simulink model "ROBOTIC_ARM_sim"  (R2024b)
settings: Solver=VariableStepAuto  StartTime=0.0  StopTime=5  RelTol=1e-3
model workspace: external: MATLAB File D:\Vaults\Mechatronic Systems Design Project\Arm\Control\robotic_arm_4dof_matlab\scripts\initalize_model.m (data not in the file)
undefined symbols (not defined in the file): cubes, sim_relative, smiData, v_b, X, Y, Z
libraries: sm_lib x75, nesl_utility x10, BUMBLEBEE x8
(part 1 of 2)
settings Model: Creator=Mohammed Hany  LastModifiedBy=Mohammed Hany

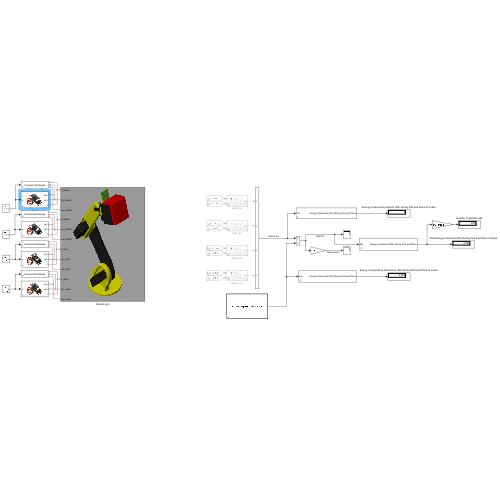
[thumbnail: Simulink's stored preview of the top-level diagram]
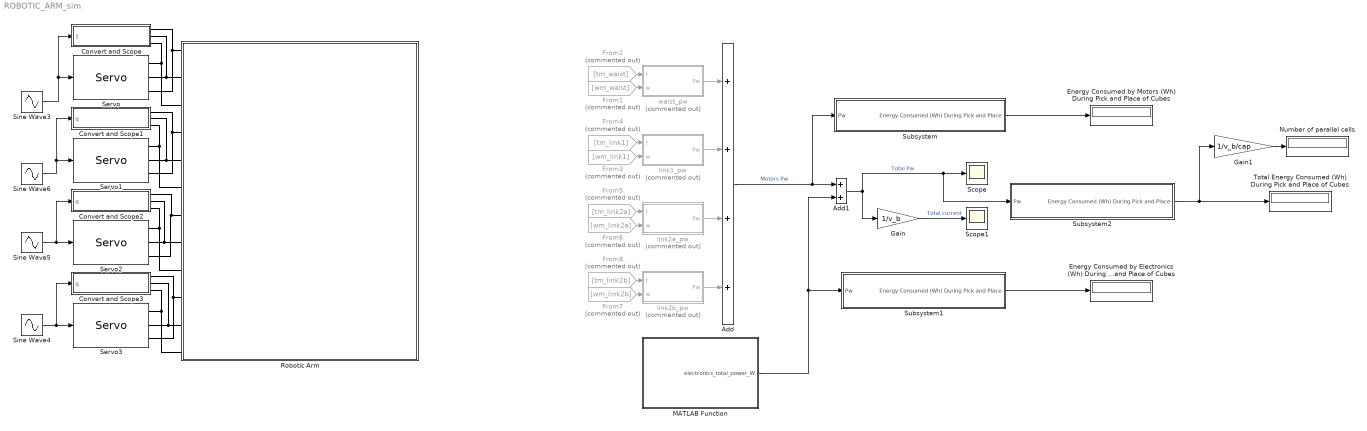
== system ROBOTIC_ARM_sim ==
  Add : Sum  Inputs=++++
  Add1 : Sum
  Convert and Scope : Subsystem  ReferencedSubsystem=convert_and_scope
      settings: PortSchema="{\"entries\":[{\"content\":{\"sides\":[{\"content\":{\"connectorIds\":[\"LConn1\",\"LConn2\"]},\"type\":\"ConnectorPlacement.EquallySpacedRectSide\",\"uuid\":\"e9d3fa8a-a658-421c-a715-dee0f5d0277a\"},{\"content\":{\"side\":\"RIGHT\"},\"type\":\"ConnectorPlacement.EquallySpacedRectSide\",\"uuid\":\"8f4733ec-a2c9-48cc-bea1-8566252d8d79\"},{\"content\":{\"connectorIds\":[\"In1\"],\"side\":\"TOP\"},\"type\":\"ConnectorPlacement.EquallySpacedRectSide\",\"uuid\":\"ce7ba2ac-a2b1-42d2-bf3f-12c1e6573af0\"},{\"content\":{\"connectorIds\":[\"RConn1\",\"RConn2\",\"RConn3\"],\"side\":\"BOTTOM\"},\"type\":\"ConnectorPlacement.EquallySpacedRectSide\",\"uuid\":\"8390652c-32f7-42bc-a6e4-5fbde262c394\"}]},\"type\":\"ConnectorPlacement.EquallySpacedConnector\",\"uuid\":\"90170afb-acac-48c1-856c-2f07de9489fa\"}],\"packageUris\":[\"http://schema.mathworks.com/mf0/Connector/R2020b\"],\"version\":\"1.0\"}"
  Convert and Scope1 : Subsystem  mask(Tool){}
      mask help: Takes the input angular position, measured angular position, measured angular velocity, torque, current, and voltage. It converts them to simulink signals and displays them on a scope. It uses a GOTO tag to cleanly expose torque, angular velocity, current, and voltage for furter computations in this model
      settings: PortSchema="{\"entries\":[{\"content\":{\"sides\":[{\"content\":{},\"type\":\"ConnectorPlacement.EquallySpacedRectSide\",\"uuid\":\"e9d3fa8a-a658-421c-a715-dee0f5d0277a\"},{\"content\":{\"side\":\"RIGHT\"},\"type\":\"ConnectorPlacement.EquallySpacedRectSide\",\"uuid\":\"8f4733ec-a2c9-48cc-bea1-8566252d8d79\"},{\"content\":{\"connectorIds\":[\"In1\"],\"side\":\"TOP\"},\"type\":\"ConnectorPlacement.EquallySpacedRectSide\",\"uuid\":\"ce7ba2ac-a2b1-42d2-bf3f-12c1e6573af0\"},{\"content\":{\"connectorIds\":[\"RConn1\",\"RConn2\",\"RConn3\"],\"side\":\"BOTTOM\"},\"type\":\"ConnectorPlacement.EquallySpacedRectSide\",\"uuid\":\"8390652c-32f7-42bc-a6e4-5fbde262c394\"}]},\"type\":\"ConnectorPlacement.EquallySpacedConnector\",\"uuid\":\"90170afb-acac-48c1-856c-2f07de9489fa\"}],\"packageUris\":[\"http://schema.mathworks.com/mf0/Connector/R2020b\"],\"version\":\"1.0\"}"
      mask Display: disp('Convert and Scope');
  Convert and Scope2 : Subsystem  mask(Tool){}
      mask help: Takes the input angular position, measured angular position, measured angular velocity, torque, current, and voltage. It converts them to simulink signals and displays them on a scope. It uses a GOTO tag to cleanly expose torque, angular velocity, current, and voltage for furter computations in this model
      settings: PortSchema="{\"entries\":[{\"content\":{\"sides\":[{\"content\":{},\"type\":\"ConnectorPlacement.EquallySpacedRectSide\",\"uuid\":\"e9d3fa8a-a658-421c-a715-dee0f5d0277a\"},{\"content\":{\"side\":\"RIGHT\"},\"type\":\"ConnectorPlacement.EquallySpacedRectSide\",\"uuid\":\"8f4733ec-a2c9-48cc-bea1-8566252d8d79\"},{\"content\":{\"connectorIds\":[\"In1\"],\"side\":\"TOP\"},\"type\":\"ConnectorPlacement.EquallySpacedRectSide\",\"uuid\":\"ce7ba2ac-a2b1-42d2-bf3f-12c1e6573af0\"},{\"content\":{\"connectorIds\":[\"RConn1\",\"RConn2\",\"RConn3\"],\"side\":\"BOTTOM\"},\"type\":\"ConnectorPlacement.EquallySpacedRectSide\",\"uuid\":\"8390652c-32f7-42bc-a6e4-5fbde262c394\"}]},\"type\":\"ConnectorPlacement.EquallySpacedConnector\",\"uuid\":\"90170afb-acac-48c1-856c-2f07de9489fa\"}],\"packageUris\":[\"http://schema.mathworks.com/mf0/Connector/R2020b\"],\"version\":\"1.0\"}"
      mask Display: disp('Convert and Scope');
  Convert and Scope3 : Subsystem  mask(Tool){}
      mask help: Takes the input angular position, measured angular position, measured angular velocity, torque, current, and voltage. It converts them to simulink signals and displays them on a scope. It uses a GOTO tag to cleanly expose torque, angular velocity, current, and voltage for furter computations in this model
      settings: PortSchema="{\"entries\":[{\"content\":{\"sides\":[{\"content\":{},\"type\":\"ConnectorPlacement.EquallySpacedRectSide\",\"uuid\":\"e9d3fa8a-a658-421c-a715-dee0f5d0277a\"},{\"content\":{\"side\":\"RIGHT\"},\"type\":\"ConnectorPlacement.EquallySpacedRectSide\",\"uuid\":\"8f4733ec-a2c9-48cc-bea1-8566252d8d79\"},{\"content\":{\"connectorIds\":[\"In1\"],\"side\":\"TOP\"},\"type\":\"ConnectorPlacement.EquallySpacedRectSide\",\"uuid\":\"ce7ba2ac-a2b1-42d2-bf3f-12c1e6573af0\"},{\"content\":{\"connectorIds\":[\"RConn1\",\"RConn2\",\"RConn3\"],\"side\":\"BOTTOM\"},\"type\":\"ConnectorPlacement.EquallySpacedRectSide\",\"uuid\":\"8390652c-32f7-42bc-a6e4-5fbde262c394\"}]},\"type\":\"ConnectorPlacement.EquallySpacedConnector\",\"uuid\":\"90170afb-acac-48c1-856c-2f07de9489fa\"}],\"packageUris\":[\"http://schema.mathworks.com/mf0/Connector/R2020b\"],\"version\":\"1.0\"}"
      mask Display: disp('Convert and Scope');
  Energy Consumed by Electronics (Wh) During Pick and Place of Cubes : Display
  Energy Consumed by Motors (Wh) During Pick and Place of Cubes : Display
  From1 : From  Commented=on  GotoTag=wm_waist
  From2 : From  Commented=on  GotoTag=tm_waist
  From3 : From  Commented=on  GotoTag=wm_link1
  From4 : From  Commented=on  GotoTag=tm_link1
  From5 : From  Commented=on  GotoTag=tm_link2a
  From6 : From  Commented=on  GotoTag=wm_link2a
  From7 : From  Commented=on  GotoTag=wm_link2b
  From8 : From  Commented=on  GotoTag=tm_link2b
  Gain : Gain  Gain=1/v_b
  Gain1 : Gain  Gain=1/v_b/cap
  MATLAB Function : MATLAB Function  TreatAsAtomicUnit=on
  Number of parallel cells : Display
  Robotic Arm : Subsystem
      mask Display: image('isometric.png');
  Scope : Scope
  Scope1 : Scope
  Servo{,1..3} (4 alike) : BUMBLEBEE/Servo  J=0 cm^2*g  La=12e-6 H  P_rated=4.2 W  V_i_noload=6 V  V_rated=6 V  i_noload=0.05 A  w_max=99 rpm  w_rated=71.43 rpm  ratio=1
  Sine Wave3 : Sin  Amplitude=55  Bias=30  SampleTime=0
  Sine Wave4 : Sin  Amplitude=180  SampleTime=0
  Sine Wave5 : Sin  Amplitude=100  Bias=-50  SampleTime=0
  Sine Wave6 : Sin  Amplitude=100  Bias=50  SampleTime=0
  Subsystem : Subsystem  mask{cubes=cubes}
      mask prompts: cubes "Number of cubes for pick and place"
  Subsystem1 : Subsystem  mask{cubes=cubes}
      mask prompts: cubes "Number of cubes for pick and place"
  Subsystem2 : Subsystem  mask{cubes=cubes}
      mask prompts: cubes "Number of cubes for pick and place"
  Total Energy Consumed (Wh) During Pick and Place of Cubes : Display
  link1_pw : Subsystem  Commented=on
  link2a_pw : Subsystem  Commented=on
  link2b_pw : Subsystem  Commented=on
  waist_pw : Subsystem  Commented=on
  wires:
  link2b_pw/1(Pw) -> Add/4
  link1_pw/1(Pw) -> Add/2
  waist_pw/1(Pw) -> Add/1
  Add/1 -> Subsystem/1(Pw), Add1/1  "Motors Pw"
  Subsystem1/1(Energy Consumed (Wh) During Pick and Place) -> Energy Consumed by Electronics (Wh) During Pick and Place of Cubes/1
  MATLAB Function/1(electronics_total_power_W) -> Add1/2, Subsystem1/1(Pw)
  Subsystem/1(Energy Consumed (Wh) During Pick and Place) -> Energy Consumed by Motors (Wh) During Pick and Place of Cubes/1
  Gain/1 -> Scope1/1  "Total current"
  Add1/1 -> Gain/1, Subsystem2/1(Pw), Scope/1  "Total Pw"
  Subsystem2/1(Energy Consumed (Wh) During Pick and Place) -> Gain1/1, Total Energy Consumed (Wh) During Pick and Place of Cubes/1
  Gain1/1 -> Number of parallel cells/1
  link2a_pw/1(Pw) -> Add/3
  Sine Wave3/1 -> Convert and Scope/1, Servo/1
  From1/1 -> waist_pw/2(w)
  From2/1 -> waist_pw/1(t)
  From4/1 -> link1_pw/1(t)
  From3/1 -> link1_pw/2(w)
  From5/1 -> link2a_pw/1(t)
  From6/1 -> link2a_pw/2(w)
  From7/1 -> link2b_pw/2(w)
  From8/1 -> link2b_pw/1(t)
  Sine Wave6/1 -> Convert and Scope1/1(q), Servo1/1
  Sine Wave5/1 -> Convert and Scope2/1(q), Servo2/1
  Sine Wave4/1 -> Convert and Scope3/1(q), Servo3/1
  connections:
  Servo/RConn2 -- Convert and Scope/RConn2 -- Robotic Arm/LConn2
  Servo/RConn1 -- Convert and Scope/RConn1 -- Robotic Arm/LConn3
  Servo1/RConn2 -- Convert and Scope1/RConn2 -- Robotic Arm/LConn5
  Servo1/RConn1 -- Convert and Scope1/RConn1 -- Robotic Arm/LConn6
  Servo1/RConn3 -- Convert and Scope1/RConn3 -- Robotic Arm/LConn4
  Servo2/RConn2 -- Convert and Scope2/RConn2 -- Robotic Arm/LConn8
  Servo2/RConn1 -- Robotic Arm/LConn9 -- Convert and Scope2/RConn1
  Servo2/RConn3 -- Convert and Scope2/RConn3 -- Robotic Arm/LConn7
  Servo3/RConn2 -- Convert and Scope3/RConn2 -- Robotic Arm/LConn11
  Servo3/RConn1 -- Convert and Scope3/RConn1 -- Robotic Arm/LConn12
  Servo3/RConn3 -- Convert and Scope3/RConn3 -- Robotic Arm/LConn10
  Servo/RConn3 -- Convert and Scope/RConn3 -- Robotic Arm/LConn1

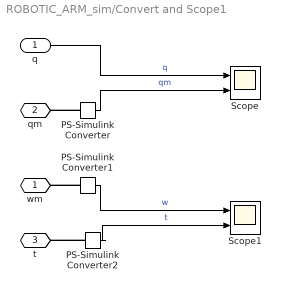
== system ROBOTIC_ARM_sim/Convert and Scope1 ==
  q : Inport
  PS-Simulink Converter : nesl_utility/PS-Simulink Converter  PhysicalDomain=network_engine_domain  SubClassName=ps_output  LeftPortType=input  RightPortType=output  PseudoPeriodic=off  Frequencies=[]  VectorFormat=inherit  Unit=deg  AffineConversion=off
  PS-Simulink Converter1 : nesl_utility/PS-Simulink Converter  PhysicalDomain=network_engine_domain  SubClassName=ps_output  LeftPortType=input  RightPortType=output  PseudoPeriodic=off  Frequencies=[]  VectorFormat=inherit  Unit=rpm  AffineConversion=off
  PS-Simulink Converter2 : nesl_utility/PS-Simulink Converter  PhysicalDomain=network_engine_domain  SubClassName=ps_output  LeftPortType=input  RightPortType=output  PseudoPeriodic=off  Frequencies=[]  VectorFormat=inherit  Unit=N*m  AffineConversion=off
  Scope : Scope  NumInputPorts=2
  Scope1 : Scope  NumInputPorts=2
  wm : PMIOPort  Side=Right
  qm : PMIOPort  Port=2  Side=Right
  t : PMIOPort  Port=3  Side=Right
  wires:
  q/1 -> Scope/1  "q"
  PS-Simulink Converter/1 -> Scope/2  "qm"
  PS-Simulink Converter2/1 -> Scope1/2  "t"
  PS-Simulink Converter1/1 -> Scope1/1  "w"
  connections:
  PS-Simulink Converter1/LConn1 -- wm/RConn1
  PS-Simulink Converter/LConn1 -- qm/RConn1
  PS-Simulink Converter2/LConn1 -- t/RConn1

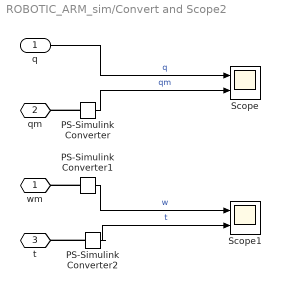
== system ROBOTIC_ARM_sim/Convert and Scope2 ==
  q : Inport
  PS-Simulink Converter : nesl_utility/PS-Simulink Converter  PhysicalDomain=network_engine_domain  SubClassName=ps_output  LeftPortType=input  RightPortType=output  PseudoPeriodic=off  Frequencies=[]  VectorFormat=inherit  Unit=deg  AffineConversion=off
  PS-Simulink Converter1 : nesl_utility/PS-Simulink Converter  PhysicalDomain=network_engine_domain  SubClassName=ps_output  LeftPortType=input  RightPortType=output  PseudoPeriodic=off  Frequencies=[]  VectorFormat=inherit  Unit=rpm  AffineConversion=off
  PS-Simulink Converter2 : nesl_utility/PS-Simulink Converter  PhysicalDomain=network_engine_domain  SubClassName=ps_output  LeftPortType=input  RightPortType=output  PseudoPeriodic=off  Frequencies=[]  VectorFormat=inherit  Unit=N*m  AffineConversion=off
  Scope : Scope  NumInputPorts=2
  Scope1 : Scope  NumInputPorts=2
  wm : PMIOPort  Side=Right
  qm : PMIOPort  Port=2  Side=Right
  t : PMIOPort  Port=3  Side=Right
  wires:
  q/1 -> Scope/1  "q"
  PS-Simulink Converter/1 -> Scope/2  "qm"
  PS-Simulink Converter2/1 -> Scope1/2  "t"
  PS-Simulink Converter1/1 -> Scope1/1  "w"
  connections:
  PS-Simulink Converter1/LConn1 -- wm/RConn1
  PS-Simulink Converter/LConn1 -- qm/RConn1
  PS-Simulink Converter2/LConn1 -- t/RConn1

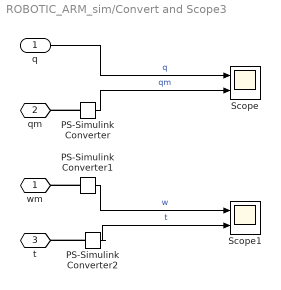
== system ROBOTIC_ARM_sim/Convert and Scope3 ==
  q : Inport
  PS-Simulink Converter : nesl_utility/PS-Simulink Converter  PhysicalDomain=network_engine_domain  SubClassName=ps_output  LeftPortType=input  RightPortType=output  PseudoPeriodic=off  Frequencies=[]  VectorFormat=inherit  Unit=deg  AffineConversion=off
  PS-Simulink Converter1 : nesl_utility/PS-Simulink Converter  PhysicalDomain=network_engine_domain  SubClassName=ps_output  LeftPortType=input  RightPortType=output  PseudoPeriodic=off  Frequencies=[]  VectorFormat=inherit  Unit=rpm  AffineConversion=off
  PS-Simulink Converter2 : nesl_utility/PS-Simulink Converter  PhysicalDomain=network_engine_domain  SubClassName=ps_output  LeftPortType=input  RightPortType=output  PseudoPeriodic=off  Frequencies=[]  VectorFormat=inherit  Unit=N*m  AffineConversion=off
  Scope : Scope  NumInputPorts=2
  Scope1 : Scope  NumInputPorts=2
  wm : PMIOPort  Side=Right
  qm : PMIOPort  Port=2  Side=Right
  t : PMIOPort  Port=3  Side=Right
  wires:
  q/1 -> Scope/1  "q"
  PS-Simulink Converter/1 -> Scope/2  "qm"
  PS-Simulink Converter2/1 -> Scope1/2  "t"
  PS-Simulink Converter1/1 -> Scope1/1  "w"
  connections:
  PS-Simulink Converter1/LConn1 -- wm/RConn1
  PS-Simulink Converter/LConn1 -- qm/RConn1
  PS-Simulink Converter2/LConn1 -- t/RConn1

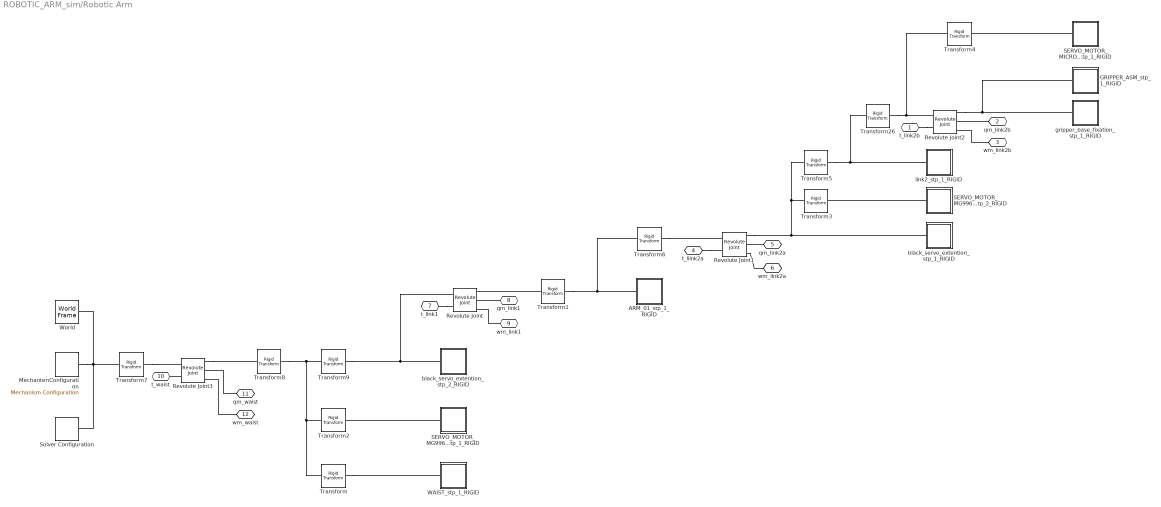
== system ROBOTIC_ARM_sim/Robotic Arm ==
  ARM_01_stp_1_RIGID : Subsystem
  GRIPPER_ASM_stp_1_RIGID : Subsystem
  MechanismConfiguration : sm_lib/Utilities/Mechanism Configuration  UniformGravity=Constant  GravityVector=[0 0 0]  GravityVectorUnits=m/s^2  LinearizationDelta=0.001  JointModeTransitionNonlinearIterations=2
  Revolute Joint{,1..3} (4 alike) : sm_lib/Joints/Revolute Joint  JointMode=Normal  CompositeWrenchDir=FollowerOnBase  CompositeWrenchFrame=BaseFrame  SenseConstraintForce=off  SenseConstraintTorque=off  SenseTotalForce=off  SenseTotalTorque=off  PositionTargetSpecify=off  PositionTargetPriority=High  PositionTargetValue=0  PositionTargetValueUnits=deg  VelocityTargetSpecify=off  VelocityTargetPriority=High  VelocityTargetValue=0  VelocityTargetValueUnits=deg/s  EquilibriumPosition=0  EquilibriumPositionUnits=deg  SpringStiffness=0  SpringStiffnessUnits=N*m/deg  DampingCoefficient=0  DampingCoefficientUnits=N*m/(deg/s)  LowerLimitSpecify=off  LowerLimitBound=-90  LowerLimitBoundUnits=deg  LowerLimitStiffness=1e4  LowerLimitStiffnessUnits=N*m/deg  LowerLimitDamping=10  LowerLimitDampingUnits=N*m/(deg/s)  LowerLimitTransitionRegionWidth=0.1  LowerLimitTransitionRegionWidthUnits=deg  UpperLimitSpecify=off  UpperLimitBound=90  UpperLimitBoundUnits=deg  UpperLimitStiffness=1e4  UpperLimitStiffnessUnits=N*m/deg  UpperLimitDamping=10  UpperLimitDampingUnits=N*m/(deg/s)  UpperLimitTransitionRegionWidth=0.1  UpperLimitTransitionRegionWidthUnits=deg  TorqueActuationMode=InputTorque  MotionActuationMode=ComputedMotion  SensePosition=on  SenseVelocity=on  SenseAcceleration=off  SenseTorqueForce=off  SenseLowerLimitTorqueForce=off  SenseUpperLimitTorqueForce=off
  SERVO_MOTOR_MG996R_stp_1_RIGID : Subsystem
  SERVO_MOTOR_MG996R_stp_2_RIGID : Subsystem
  SERVO_MOTOR_MICRO_9G_stp_1_RIGID : Subsystem
  Solver Configuration : nesl_utility/Solver Configuration  PhysicalDomain=network_engine_domain  SubClassName=solver  LeftPortType=input  RightPortType=generic  Tones=[]  Harmonics=[]  SimulateNoise=off  Profile=off  UseLocalSampling=off  EnableSwitchedLinearOptims=on  FrequencyDomain=off  UseCCode=off  RelTol=0.001  AbsTol=0.001  MinStep=1e-09  ToWorkspace=off  RevertToSquareIcSolve=off  NumHomotopyIterations=100  PhasorMode=off  PhasorModeNumHarmonics=1  ConsistencySolver=NEWTON_XTOL_AFTER_FTOL  IndexReductionMethod=DerivativeReplacement  DoDC=off  ResidualTolerance=1e-09  ConsistencyTolSource=GLOBAL  ConsistencyAbsTol=0.001  ConsistencyRelTol=0.001  ConsistencyTolFactor=0.001  UseLocalSolver=off  LocalSolverChoice=NE_BACKWARD_EULER_ADVANCER  ResolveIndetEquations=on  FunctionEvalNumThread=1  LocalSolverSampleTime=0.001  DoFixedCost=off  MaxNonlinIter=3  MaxModeIter=2  ComputeImpulses=off  ImpulseIterations=2  LinearAlgebra=auto  LinearAlgebraNumThread=0  EquationFormulation=NE_TIME_EF  DelaysMemoryBudget=1024  AutomaticFiltering=on  FilteringTimeConstant=0.001  PartitionStorageMethod=AS_NEEDED  PartitionMemoryBudget=1024  PartitionMethod=ROBUST  MultibodyUseLocalSolver=off  MultibodyLocalSolverChoice=ODE1  MultibodyLocalSolverSampleTime=0.001
  Transform : sm_lib/Frames and Transforms/Rigid Transform  RotationMethod=ArbitraryAxis  FollAlignAxisA=+X  BaseAlignAxisA=+Y  FollAlignAxisB=+Y  BaseAlignAxisB=+Z  RotationStandardAxis=+Z  RotationAngle=smiData.RigidTransform(25).angle  RotationAngleUnits=rad  RotationArbitraryAxis=smiData.RigidTransform(25).axis  RotationSequenceAxes=FollowerAxes  RotationSequence=XYX  RotationSequenceAngles=[0 0 0]  RotationSequenceAnglesUnits=deg  RotationMatrix=[1 0 0;0 1 0;0 0 1]  Quaternion=[1 0 0 0]  TranslationMethod=Cartesian  TranslationCartesianOffset=smiData.RigidTransform(25).translation  TranslationCartesianOffsetUnits=mm  TranslationStandardAxis=+Z  TranslationStandardOffset=0  TranslationStandardOffsetUnits=m  TranslationROffset=0  TranslationROffsetUnits=m  TranslationThetaOffset=0  TranslationThetaOffsetUnits=deg  TranslationZOffset=0  TranslationZOffsetUnits=m
  Transform1 : sm_lib/Frames and Transforms/Rigid Transform  RotationMethod=ArbitraryAxis  FollAlignAxisA=+X  BaseAlignAxisA=+Y  FollAlignAxisB=+Y  BaseAlignAxisB=+Z  RotationStandardAxis=+Z  RotationAngle=sim_relative(1).angle  RotationAngleUnits=rad  RotationArbitraryAxis=sim_relative(1).axis  RotationSequenceAxes=FollowerAxes  RotationSequence=XYX  RotationSequenceAngles=[0 0 0]  RotationSequenceAnglesUnits=deg  RotationMatrix=[1 0 0;0 1 0;0 0 1]  Quaternion=[1 0 0 0]  TranslationMethod=Cartesian  TranslationCartesianOffset=sim_relative(1).translation  TranslationCartesianOffsetUnits=mm  TranslationStandardAxis=+Z  TranslationStandardOffset=0  TranslationStandardOffsetUnits=m  TranslationROffset=0  TranslationROffsetUnits=m  TranslationThetaOffset=0  TranslationThetaOffsetUnits=deg  TranslationZOffset=0  TranslationZOffsetUnits=m
  Transform2 : sm_lib/Frames and Transforms/Rigid Transform  RotationMethod=ArbitraryAxis  FollAlignAxisA=+X  BaseAlignAxisA=+Y  FollAlignAxisB=+Y  BaseAlignAxisB=+Z  RotationStandardAxis=+Z  RotationAngle=smiData.RigidTransform(27).angle  RotationAngleUnits=rad  RotationArbitraryAxis=smiData.RigidTransform(27).axis  RotationSequenceAxes=FollowerAxes  RotationSequence=XYX  RotationSequenceAngles=[0 0 0]  RotationSequenceAnglesUnits=deg  RotationMatrix=[1 0 0;0 1 0;0 0 1]  Quaternion=[1 0 0 0]  TranslationMethod=Cartesian  TranslationCartesianOffset=smiData.RigidTransform(27).translation  TranslationCartesianOffsetUnits=mm  TranslationStandardAxis=+Z  TranslationStandardOffset=0  TranslationStandardOffsetUnits=m  TranslationROffset=0  TranslationROffsetUnits=m  TranslationThetaOffset=0  TranslationThetaOffsetUnits=deg  TranslationZOffset=0  TranslationZOffsetUnits=m
  Transform26 : sm_lib/Frames and Transforms/Rigid Transform  RotationMethod=ArbitraryAxis  FollAlignAxisA=+X  BaseAlignAxisA=+Y  FollAlignAxisB=+Y  BaseAlignAxisB=+Z  RotationStandardAxis=+Z  RotationAngle=sim_relative(5).angle  RotationAngleUnits=rad  RotationArbitraryAxis=sim_relative(5).axis  RotationSequenceAxes=FollowerAxes  RotationSequence=XYX  RotationSequenceAngles=[0 0 0]  RotationSequenceAnglesUnits=deg  RotationMatrix=[1 0 0;0 1 0;0 0 1]  Quaternion=[1 0 0 0]  TranslationMethod=Cartesian  TranslationCartesianOffset=sim_relative(5).translation  TranslationCartesianOffsetUnits=mm  TranslationStandardAxis=+Z  TranslationStandardOffset=0  TranslationStandardOffsetUnits=m  TranslationROffset=0  TranslationROffsetUnits=m  TranslationThetaOffset=0  TranslationThetaOffsetUnits=deg  TranslationZOffset=0  TranslationZOffsetUnits=m
  Transform3 : sm_lib/Frames and Transforms/Rigid Transform  RotationMethod=ArbitraryAxis  FollAlignAxisA=+X  BaseAlignAxisA=+Y  FollAlignAxisB=+Y  BaseAlignAxisB=+Z  RotationStandardAxis=+Z  RotationAngle=sim_relative(4).angle  RotationAngleUnits=rad  RotationArbitraryAxis=sim_relative(4).axis  RotationSequenceAxes=FollowerAxes  RotationSequence=XYX  RotationSequenceAngles=[0 0 0]  RotationSequenceAnglesUnits=deg  RotationMatrix=[1 0 0;0 1 0;0 0 1]  Quaternion=[1 0 0 0]  TranslationMethod=Cartesian  TranslationCartesianOffset=sim_relative(4).translation  TranslationCartesianOffsetUnits=mm  TranslationStandardAxis=+Z  TranslationStandardOffset=0  TranslationStandardOffsetUnits=m  TranslationROffset=0  TranslationROffsetUnits=m  TranslationThetaOffset=0  TranslationThetaOffsetUnits=deg  TranslationZOffset=0  TranslationZOffsetUnits=m
  Transform4 : sm_lib/Frames and Transforms/Rigid Transform  RotationMethod=ArbitraryAxis  FollAlignAxisA=+X  BaseAlignAxisA=+Y  FollAlignAxisB=+Y  BaseAlignAxisB=+Z  RotationStandardAxis=+Z  RotationAngle=sim_relative(8).angle  RotationAngleUnits=rad  RotationArbitraryAxis=sim_relative(8).axis  RotationSequenceAxes=FollowerAxes  RotationSequence=XYX  RotationSequenceAngles=[0 0 0]  RotationSequenceAnglesUnits=deg  RotationMatrix=[1 0 0;0 1 0;0 0 1]  Quaternion=[1 0 0 0]  TranslationMethod=Cartesian  TranslationCartesianOffset=sim_relative(8).translation  TranslationCartesianOffsetUnits=mm  TranslationStandardAxis=+Z  TranslationStandardOffset=0  TranslationStandardOffsetUnits=m  TranslationROffset=0  TranslationROffsetUnits=m  TranslationThetaOffset=0  TranslationThetaOffsetUnits=deg  TranslationZOffset=0  TranslationZOffsetUnits=m
  Transform5 : sm_lib/Frames and Transforms/Rigid Transform  RotationMethod=ArbitraryAxis  FollAlignAxisA=+X  BaseAlignAxisA=+Y  FollAlignAxisB=+Y  BaseAlignAxisB=+Z  RotationStandardAxis=+Z  RotationAngle=sim_relative(6).angle  RotationAngleUnits=rad  RotationArbitraryAxis=sim_relative(6).axis  RotationSequenceAxes=FollowerAxes  RotationSequence=XYX  RotationSequenceAngles=[0 0 0]  RotationSequenceAnglesUnits=deg  RotationMatrix=[1 0 0;0 1 0;0 0 1]  Quaternion=[1 0 0 0]  TranslationMethod=Cartesian  TranslationCartesianOffset=sim_relative(6).translation  TranslationCartesianOffsetUnits=mm  TranslationStandardAxis=+Z  TranslationStandardOffset=0  TranslationStandardOffsetUnits=m  TranslationROffset=0  TranslationROffsetUnits=m  TranslationThetaOffset=0  TranslationThetaOffsetUnits=deg  TranslationZOffset=0  TranslationZOffsetUnits=m
  Transform6 : sm_lib/Frames and Transforms/Rigid Transform  RotationMethod=ArbitraryAxis  FollAlignAxisA=+X  BaseAlignAxisA=+Y  FollAlignAxisB=+Y  BaseAlignAxisB=+Z  RotationStandardAxis=+Z  RotationAngle=sim_relative(3).angle  RotationAngleUnits=rad  RotationArbitraryAxis=sim_relative(3).axis  RotationSequenceAxes=FollowerAxes  RotationSequence=XYX  RotationSequenceAngles=[0 0 0]  RotationSequenceAnglesUnits=deg  RotationMatrix=[1 0 0;0 1 0;0 0 1]  Quaternion=[1 0 0 0]  TranslationMethod=Cartesian  TranslationCartesianOffset=sim_relative(3).translation  TranslationCartesianOffsetUnits=mm  TranslationStandardAxis=+Z  TranslationStandardOffset=0  TranslationStandardOffsetUnits=m  TranslationROffset=0  TranslationROffsetUnits=m  TranslationThetaOffset=0  TranslationThetaOffsetUnits=deg  TranslationZOffset=0  TranslationZOffsetUnits=m
  Transform7 : sm_lib/Frames and Transforms/Rigid Transform  RotationMethod=None  FollAlignAxisA=+X  BaseAlignAxisA=+Y  FollAlignAxisB=+Y  BaseAlignAxisB=+Z  RotationStandardAxis=+X  RotationAngle=pi/2  RotationAngleUnits=rad  RotationArbitraryAxis=smiData.RigidTransform(63).axis  RotationSequenceAxes=FollowerAxes  RotationSequence=XYX  RotationSequenceAngles=[0 0 0]  RotationSequenceAnglesUnits=deg  RotationMatrix=[1 0 0;0 1 0;0 0 1]  Quaternion=[1 0 0 0]  TranslationMethod=Cartesian  TranslationCartesianOffset=smiData.RigidTransform(63).translation  TranslationCartesianOffsetUnits=mm  TranslationStandardAxis=+Z  TranslationStandardOffset=0  TranslationStandardOffsetUnits=m  TranslationROffset=0  TranslationROffsetUnits=m  TranslationThetaOffset=0  TranslationThetaOffsetUnits=deg  TranslationZOffset=0  TranslationZOffsetUnits=m
  Transform8 : sm_lib/Frames and Transforms/Rigid Transform  RotationMethod=StandardAxis  FollAlignAxisA=+X  BaseAlignAxisA=+Y  FollAlignAxisB=+Y  BaseAlignAxisB=+Z  RotationStandardAxis=+X  RotationAngle=pi/2  RotationAngleUnits=rad  RotationArbitraryAxis=smiData.RigidTransform(63).axis  RotationSequenceAxes=FollowerAxes  RotationSequence=XYX  RotationSequenceAngles=[0 0 0]  RotationSequenceAnglesUnits=deg  RotationMatrix=[1 0 0;0 1 0;0 0 1]  Quaternion=[1 0 0 0]  TranslationMethod=Cartesian  TranslationCartesianOffset=smiData.RigidTransform(63).translation  TranslationCartesianOffsetUnits=mm  TranslationStandardAxis=+Z  TranslationStandardOffset=0  TranslationStandardOffsetUnits=m  TranslationROffset=0  TranslationROffsetUnits=m  TranslationThetaOffset=0  TranslationThetaOffsetUnits=deg  TranslationZOffset=0  TranslationZOffsetUnits=m
  Transform9 : sm_lib/Frames and Transforms/Rigid Transform  RotationMethod=ArbitraryAxis  FollAlignAxisA=+X  BaseAlignAxisA=+Y  FollAlignAxisB=+Y  BaseAlignAxisB=+Z  RotationStandardAxis=+Z  RotationAngle=smiData.RigidTransform(34).angle  RotationAngleUnits=rad  RotationArbitraryAxis=smiData.RigidTransform(34).axis  RotationSequenceAxes=FollowerAxes  RotationSequence=XYX  RotationSequenceAngles=[0 0 0]  RotationSequenceAnglesUnits=deg  RotationMatrix=[1 0 0;0 1 0;0 0 1]  Quaternion=[1 0 0 0]  TranslationMethod=Cartesian  TranslationCartesianOffset=smiData.RigidTransform(34).translation  TranslationCartesianOffsetUnits=mm  TranslationStandardAxis=+Z  TranslationStandardOffset=0  TranslationStandardOffsetUnits=m  TranslationROffset=0  TranslationROffsetUnits=m  TranslationThetaOffset=0  TranslationThetaOffsetUnits=deg  TranslationZOffset=0  TranslationZOffsetUnits=m
  WAIST_stp_1_RIGID : Subsystem
  World : sm_lib/Frames and Transforms/World Frame
  black_servo_extention_stp_1_RIGID : Subsystem
  black_servo_extention_stp_2_RIGID : Subsystem
  gripper_base_fixation_stp_1_RIGID : Subsystem
  link2_stp_1_RIGID : Subsystem
  t_link2b : PMIOPort  Side=Left
  qm_link2b : PMIOPort  Port=2  Side=Left
  wm_link2b : PMIOPort  Port=3  Side=Left
  t_lilnk2a : PMIOPort  Port=4  Side=Left
  qm_link2a : PMIOPort  Port=5  Side=Left
  wm_link2a : PMIOPort  Port=6  Side=Left
  t_link1 : PMIOPort  Port=7  Side=Left
  qm_link1 : PMIOPort  Port=8  Side=Left
  wm_link1 : PMIOPort  Port=9  Side=Left
  t_waist : PMIOPort  Port=10  Side=Left
  qm_waist : PMIOPort  Port=11  Side=Left
  wm_waist : PMIOPort  Port=12  Side=Left
  connections:
  Transform/RConn1 -- WAIST_stp_1_RIGID/LConn1
  Transform9/LConn1 -- Transform2/LConn1 -- Transform/LConn1 -- Transform8/RConn1
  Transform9/RConn1 -- Revolute Joint/LConn1 -- black_servo_extention_stp_2_RIGID/LConn1
  SERVO_MOTOR_MG996R_stp_1_RIGID/LConn1 -- Transform2/RConn1
  Transform1/RConn1 -- Transform6/LConn1 -- ARM_01_stp_1_RIGID/LConn1
  Transform1/LConn1 -- Revolute Joint/RConn1
  Revolute Joint2/RConn1 -- GRIPPER_ASM_stp_1_RIGID/RConn1 -- gripper_base_fixation_stp_1_RIGID/LConn1
  SERVO_MOTOR_MG996R_stp_2_RIGID/LConn1 -- Transform3/RConn1
  Transform5/RConn1 -- Transform26/LConn1 -- link2_stp_1_RIGID/LConn1
  Transform6/RConn1 -- Revolute Joint1/LConn1
  Revolute Joint1/RConn1 -- Transform5/LConn1 -- Transform3/LConn1 -- black_servo_extention_stp_1_RIGID/LConn1
  Transform26/RConn1 -- Transform4/LConn1 -- Revolute Joint2/LConn1
  SERVO_MOTOR_MICRO_9G_stp_1_RIGID/LConn1 -- Transform4/RConn1
  World/RConn1 -- MechanismConfiguration/RConn1 -- Solver Configuration/RConn1 -- Transform7/LConn1
  Transform7/RConn1 -- Revolute Joint3/LConn1
  Revolute Joint3/LConn2 -- t_waist/RConn1
  t_link2b/RConn1 -- Revolute Joint2/LConn2
  Revolute Joint3/RConn1 -- Transform8/LConn1
  wm_waist/RConn1 -- Revolute Joint3/RConn3
  qm_waist/RConn1 -- Revolute Joint3/RConn2
  t_lilnk2a/RConn1 -- Revolute Joint1/LConn2
  qm_link2a/RConn1 -- Revolute Joint1/RConn2
  wm_link2a/RConn1 -- Revolute Joint1/RConn3
  wm_link2b/RConn1 -- Revolute Joint2/RConn3
  qm_link2b/RConn1 -- Revolute Joint2/RConn2
  t_link1/RConn1 -- Revolute Joint/LConn2
  qm_link1/RConn1 -- Revolute Joint/RConn2
  wm_link1/RConn1 -- Revolute Joint/RConn3

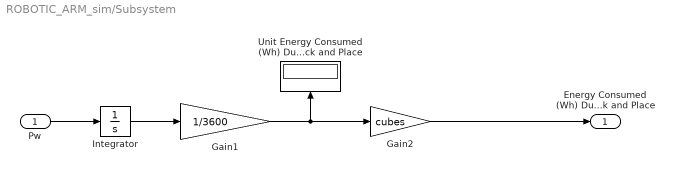
== system ROBOTIC_ARM_sim/Subsystem ==
  Pw : Inport
  Gain1 : Gain  Gain=1/3600
  Gain2 : Gain  Gain=cubes
  Integrator : Integrator
  Unit Energy Consumed (Wh) During Pick and Place : Display
  Energy Consumed (Wh) During Pick and Place : Outport
  wires:
  Integrator/1 -> Gain1/1
  Gain1/1 -> Gain2/1, Unit Energy Consumed (Wh) During Pick and Place/1
  Gain2/1 -> Energy Consumed (Wh) During Pick and Place/1
  Pw/1 -> Integrator/1

== system ROBOTIC_ARM_sim/Subsystem1 ==
  Pw : Inport
  Gain1 : Gain  Gain=1/3600
  Gain2 : Gain  Gain=cubes
  Integrator : Integrator
  Unit Energy Consumed (Wh) During Pick and Place : Display
  Energy Consumed (Wh) During Pick and Place : Outport
  wires:
  Integrator/1 -> Gain1/1
  Gain1/1 -> Gain2/1, Unit Energy Consumed (Wh) During Pick and Place/1
  Gain2/1 -> Energy Consumed (Wh) During Pick and Place/1
  Pw/1 -> Integrator/1

== system ROBOTIC_ARM_sim/Subsystem2 ==
  Pw : Inport
  Gain1 : Gain  Gain=1/3600
  Gain2 : Gain  Gain=cubes
  Integrator : Integrator
  Unit Energy Consumed (Wh) During Pick and Place : Display
  Energy Consumed (Wh) During Pick and Place : Outport
  wires:
  Integrator/1 -> Gain1/1
  Gain1/1 -> Gain2/1, Unit Energy Consumed (Wh) During Pick and Place/1
  Gain2/1 -> Energy Consumed (Wh) During Pick and Place/1
  Pw/1 -> Integrator/1

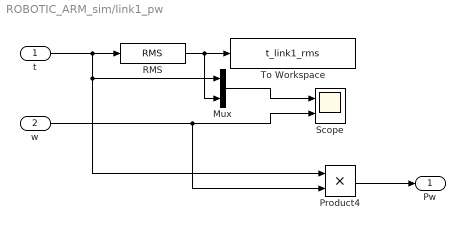
== system ROBOTIC_ARM_sim/link1_pw ==
  t : Inport
  w : Inport  Port=2
  Mux : Mux  Inputs=2
  Product4 : Product
  RMS : BUMBLEBEE/RMS
  Scope : Scope  NumInputPorts=2
  To Workspace : ToWorkspace  VariableName=t_link1_rms  SampleTime=-1
      settings: MaxDataPoints=1  Save2DSignal=2-D array (concatenate along first dimension)
  Pw : Outport
  wires:
  w/1 -> Product4/2, Scope/2
  t/1 -> RMS/1, Product4/1, Mux/1
  RMS/1 -> Mux/2, To Workspace/1
  Product4/1 -> Pw/1
  Mux/1 -> Scope/1

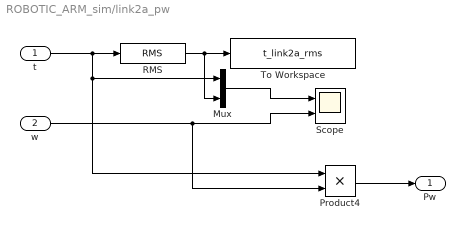
== system ROBOTIC_ARM_sim/link2a_pw ==
  t : Inport
  w : Inport  Port=2
  Mux : Mux  Inputs=2
  Product4 : Product
  RMS : BUMBLEBEE/RMS
  Scope : Scope  NumInputPorts=2
  To Workspace : ToWorkspace  VariableName=t_link2a_rms  SampleTime=-1
      settings: MaxDataPoints=1  Save2DSignal=2-D array (concatenate along first dimension)
  Pw : Outport
  wires:
  w/1 -> Product4/2, Scope/2
  t/1 -> RMS/1, Product4/1, Mux/1
  RMS/1 -> Mux/2, To Workspace/1
  Product4/1 -> Pw/1
  Mux/1 -> Scope/1

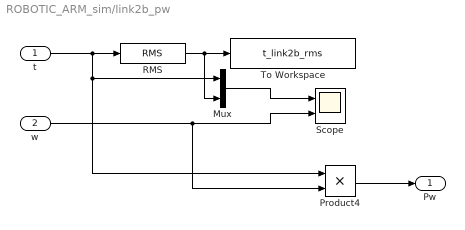
== system ROBOTIC_ARM_sim/link2b_pw ==
  t : Inport
  w : Inport  Port=2
  Mux : Mux  Inputs=2
  Product4 : Product
  RMS : BUMBLEBEE/RMS
  Scope : Scope  NumInputPorts=2
  To Workspace : ToWorkspace  VariableName=t_link2b_rms  SampleTime=-1
      settings: MaxDataPoints=1  Save2DSignal=2-D array (concatenate along first dimension)
  Pw : Outport
  wires:
  w/1 -> Product4/2, Scope/2
  t/1 -> RMS/1, Product4/1, Mux/1
  RMS/1 -> Mux/2, To Workspace/1
  Product4/1 -> Pw/1
  Mux/1 -> Scope/1

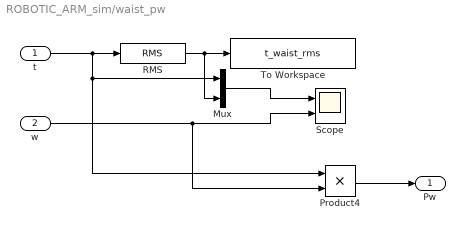
== system ROBOTIC_ARM_sim/waist_pw ==
  t : Inport
  w : Inport  Port=2
  Mux : Mux  Inputs=2
  Product4 : Product
  RMS : BUMBLEBEE/RMS
  Scope : Scope  NumInputPorts=2
  To Workspace : ToWorkspace  VariableName=t_waist_rms  SampleTime=-1
      settings: MaxDataPoints=1  Save2DSignal=2-D array (concatenate along first dimension)
  Pw : Outport
  wires:
  w/1 -> Product4/2, Scope/2
  t/1 -> RMS/1, Product4/1, Mux/1
  RMS/1 -> Mux/2, To Workspace/1
  Product4/1 -> Pw/1
  Mux/1 -> Scope/1

== system ROBOTIC_ARM_sim/Robotic Arm/ARM_01_stp_1_RIGID ==
  ReferenceFrame : sm_lib/Frames and Transforms/Reference Frame
  Solid : sm_lib/Body Elements/File Solid  ExtGeomFileName=ARM 01.stp_Default_sldprt.STEP  UnitType=FromFile  ExtGeomFileUnits=m  StepReaderType=HEX  ExportConvexHullGeometry=off  InertiaType=Custom  BasedOnType=DensityFromFile  Density=1000  DensityUnits=kg/m^3  Mass=smiData.Solid(15).mass  MassUnits=kg  CenterOfMass=smiData.Solid(15).CoM  CenterOfMassUnits=mm  MomentsOfInertia=smiData.Solid(15).MoI  MomentsOfInertiaUnits=kg*mm^2  ProductsOfInertia=smiData.Solid(15).PoI  ProductsOfInertiaUnits=kg*mm^2  GraphicType=FromGeometry  MarkerShape=Sphere  MarkerSize=10  GraphicVisPropType=SimpleVisualProperties  GraphicDiffuseColor=[0.149 0.149 0.149]  GraphicOpacity=smiData.Solid(15).opacity  GraphicSpecularColor=[0.5 0.5 0.5 1.0]  GraphicAmbientColor=[0.15 0.15 0.15 1.0]  GraphicEmissiveColor=[0.0 0.0 0.0 1.0]  GraphicShininess=75  DoExposeReferenceFrame=on  SerializedFrames=<Frames/>
  F : PMIOPort  Side=Left
  connections:
  ReferenceFrame/RConn1 -- Solid/RConn1 -- F/RConn1

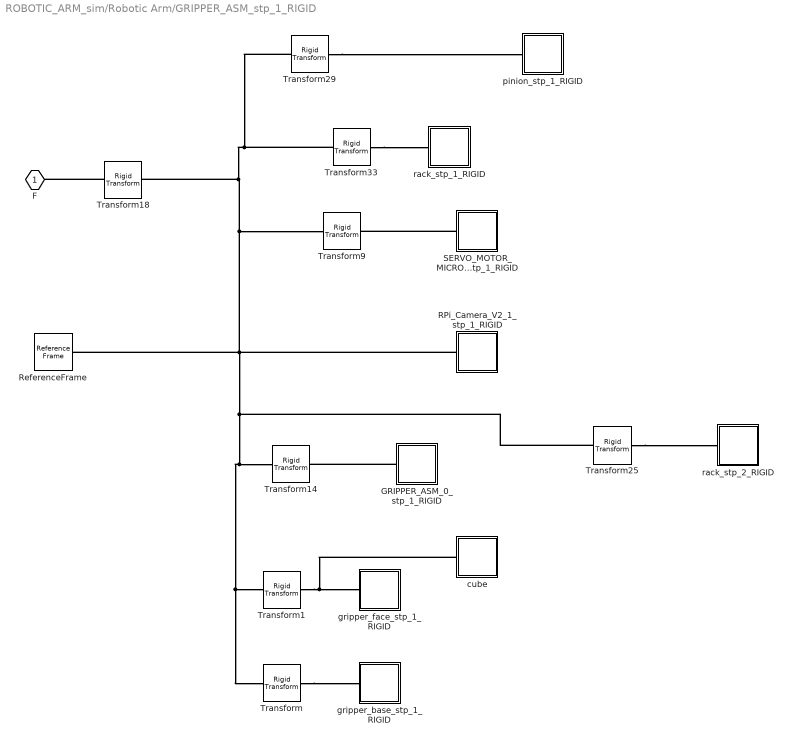
== system ROBOTIC_ARM_sim/Robotic Arm/GRIPPER_ASM_stp_1_RIGID ==
  GRIPPER_ASM_0_stp_1_RIGID : Subsystem
  RPi_Camera_V2_1_stp_1_RIGID : Subsystem
  ReferenceFrame : sm_lib/Frames and Transforms/Reference Frame
  SERVO_MOTOR_MICRO_9G_stp_1_RIGID : Subsystem
  Transform : sm_lib/Frames and Transforms/Rigid Transform  RotationMethod=ArbitraryAxis  FollAlignAxisA=+X  BaseAlignAxisA=+Y  FollAlignAxisB=+Y  BaseAlignAxisB=+Z  RotationStandardAxis=+Z  RotationAngle=smiData.RigidTransform(1).angle  RotationAngleUnits=rad  RotationArbitraryAxis=smiData.RigidTransform(1).axis  RotationSequenceAxes=FollowerAxes  RotationSequence=XYX  RotationSequenceAngles=[0 0 0]  RotationSequenceAnglesUnits=deg  RotationMatrix=[1 0 0;0 1 0;0 0 1]  Quaternion=[1 0 0 0]  TranslationMethod=Cartesian  TranslationCartesianOffset=smiData.RigidTransform(1).translation  TranslationCartesianOffsetUnits=mm  TranslationStandardAxis=+Z  TranslationStandardOffset=0  TranslationStandardOffsetUnits=m  TranslationROffset=0  TranslationROffsetUnits=m  TranslationThetaOffset=0  TranslationThetaOffsetUnits=deg  TranslationZOffset=0  TranslationZOffsetUnits=m
  Transform1 : sm_lib/Frames and Transforms/Rigid Transform  RotationMethod=ArbitraryAxis  FollAlignAxisA=+X  BaseAlignAxisA=+Y  FollAlignAxisB=+Y  BaseAlignAxisB=+Z  RotationStandardAxis=+Z  RotationAngle=smiData.RigidTransform(7).angle  RotationAngleUnits=rad  RotationArbitraryAxis=smiData.RigidTransform(7).axis  RotationSequenceAxes=FollowerAxes  RotationSequence=XYX  RotationSequenceAngles=[0 0 0]  RotationSequenceAnglesUnits=deg  RotationMatrix=[1 0 0;0 1 0;0 0 1]  Quaternion=[1 0 0 0]  TranslationMethod=Cartesian  TranslationCartesianOffset=smiData.RigidTransform(7).translation  TranslationCartesianOffsetUnits=mm  TranslationStandardAxis=+Z  TranslationStandardOffset=0  TranslationStandardOffsetUnits=m  TranslationROffset=0  TranslationROffsetUnits=m  TranslationThetaOffset=0  TranslationThetaOffsetUnits=deg  TranslationZOffset=0  TranslationZOffsetUnits=m
  Transform14 : sm_lib/Frames and Transforms/Rigid Transform  RotationMethod=ArbitraryAxis  FollAlignAxisA=+X  BaseAlignAxisA=+Y  FollAlignAxisB=+Y  BaseAlignAxisB=+Z  RotationStandardAxis=+Z  RotationAngle=smiData.RigidTransform(20).angle  RotationAngleUnits=rad  RotationArbitraryAxis=smiData.RigidTransform(20).axis  RotationSequenceAxes=FollowerAxes  RotationSequence=XYX  RotationSequenceAngles=[0 0 0]  RotationSequenceAnglesUnits=deg  RotationMatrix=[1 0 0;0 1 0;0 0 1]  Quaternion=[1 0 0 0]  TranslationMethod=Cartesian  TranslationCartesianOffset=smiData.RigidTransform(20).translation  TranslationCartesianOffsetUnits=mm  TranslationStandardAxis=+Z  TranslationStandardOffset=0  TranslationStandardOffsetUnits=m  TranslationROffset=0  TranslationROffsetUnits=m  TranslationThetaOffset=0  TranslationThetaOffsetUnits=deg  TranslationZOffset=0  TranslationZOffsetUnits=m
  Transform18 : sm_lib/Frames and Transforms/Rigid Transform  RotationMethod=ArbitraryAxis  FollAlignAxisA=+X  BaseAlignAxisA=+Y  FollAlignAxisB=+Y  BaseAlignAxisB=+Z  RotationStandardAxis=+Z  RotationAngle=sim_relative(7).angle  RotationAngleUnits=rad  RotationArbitraryAxis=sim_relative(7).axis  RotationSequenceAxes=FollowerAxes  RotationSequence=XYX  RotationSequenceAngles=[0 0 0]  RotationSequenceAnglesUnits=deg  RotationMatrix=[1 0 0;0 1 0;0 0 1]  Quaternion=[1 0 0 0]  TranslationMethod=Cartesian  TranslationCartesianOffset=sim_relative(7).translation  TranslationCartesianOffsetUnits=mm  TranslationStandardAxis=+Z  TranslationStandardOffset=0  TranslationStandardOffsetUnits=m  TranslationROffset=0  TranslationROffsetUnits=m  TranslationThetaOffset=0  TranslationThetaOffsetUnits=deg  TranslationZOffset=0  TranslationZOffsetUnits=m
  Transform25 : sm_lib/Frames and Transforms/Rigid Transform  RotationMethod=ArbitraryAxis  FollAlignAxisA=+X  BaseAlignAxisA=+Y  FollAlignAxisB=+Y  BaseAlignAxisB=+Z  RotationStandardAxis=+Z  RotationAngle=sim_relative(10).angle  RotationAngleUnits=rad  RotationArbitraryAxis=sim_relative(10).axis  RotationSequenceAxes=FollowerAxes  RotationSequence=XYX  RotationSequenceAngles=[0 0 0]  RotationSequenceAnglesUnits=deg  RotationMatrix=[1 0 0;0 1 0;0 0 1]  Quaternion=[1 0 0 0]  TranslationMethod=Cartesian  TranslationCartesianOffset=sim_relative(10).translation  TranslationCartesianOffsetUnits=mm  TranslationStandardAxis=+Z  TranslationStandardOffset=0  TranslationStandardOffsetUnits=m  TranslationROffset=0  TranslationROffsetUnits=m  TranslationThetaOffset=0  TranslationThetaOffsetUnits=deg  TranslationZOffset=0  TranslationZOffsetUnits=m
  Transform29 : sm_lib/Frames and Transforms/Rigid Transform  RotationMethod=ArbitraryAxis  FollAlignAxisA=+X  BaseAlignAxisA=+Y  FollAlignAxisB=+Y  BaseAlignAxisB=+Z  RotationStandardAxis=+Z  RotationAngle=sim_relative(11).angle  RotationAngleUnits=rad  RotationArbitraryAxis=sim_relative(11).axis  RotationSequenceAxes=FollowerAxes  RotationSequence=XYX  RotationSequenceAngles=[0 0 0]  RotationSequenceAnglesUnits=deg  RotationMatrix=[1 0 0;0 1 0;0 0 1]  Quaternion=[1 0 0 0]  TranslationMethod=Cartesian  TranslationCartesianOffset=sim_relative(11).translation  TranslationCartesianOffsetUnits=mm  TranslationStandardAxis=+Z  TranslationStandardOffset=0  TranslationStandardOffsetUnits=m  TranslationROffset=0  TranslationROffsetUnits=m  TranslationThetaOffset=0  TranslationThetaOffsetUnits=deg  TranslationZOffset=0  TranslationZOffsetUnits=m
  Transform33 : sm_lib/Frames and Transforms/Rigid Transform  RotationMethod=ArbitraryAxis  FollAlignAxisA=+X  BaseAlignAxisA=+Y  FollAlignAxisB=+Y  BaseAlignAxisB=+Z  RotationStandardAxis=+Z  RotationAngle=sim_relative(9).angle  RotationAngleUnits=rad  RotationArbitraryAxis=sim_relative(9).axis  RotationSequenceAxes=FollowerAxes  RotationSequence=XYX  RotationSequenceAngles=[0 0 0]  RotationSequenceAnglesUnits=deg  RotationMatrix=[1 0 0;0 1 0;0 0 1]  Quaternion=[1 0 0 0]  TranslationMethod=Cartesian  TranslationCartesianOffset=sim_relative(9).translation  TranslationCartesianOffsetUnits=mm  TranslationStandardAxis=+Z  TranslationStandardOffset=0  TranslationStandardOffsetUnits=m  TranslationROffset=0  TranslationROffsetUnits=m  TranslationThetaOffset=0  TranslationThetaOffsetUnits=deg  TranslationZOffset=0  TranslationZOffsetUnits=m
  Transform9 : sm_lib/Frames and Transforms/Rigid Transform  RotationMethod=ArbitraryAxis  FollAlignAxisA=+X  BaseAlignAxisA=+Y  FollAlignAxisB=+Y  BaseAlignAxisB=+Z  RotationStandardAxis=+Z  RotationAngle=smiData.RigidTransform(15).angle  RotationAngleUnits=rad  RotationArbitraryAxis=smiData.RigidTransform(15).axis  RotationSequenceAxes=FollowerAxes  RotationSequence=XYX  RotationSequenceAngles=[0 0 0]  RotationSequenceAnglesUnits=deg  RotationMatrix=[1 0 0;0 1 0;0 0 1]  Quaternion=[1 0 0 0]  TranslationMethod=Cartesian  TranslationCartesianOffset=smiData.RigidTransform(15).translation  TranslationCartesianOffsetUnits=mm  TranslationStandardAxis=+Z  TranslationStandardOffset=0  TranslationStandardOffsetUnits=m  TranslationROffset=0  TranslationROffsetUnits=m  TranslationThetaOffset=0  TranslationThetaOffsetUnits=deg  TranslationZOffset=0  TranslationZOffsetUnits=m
  cube : Subsystem
  gripper_base_stp_1_RIGID : Subsystem
  gripper_face_stp_1_RIGID : Subsystem
  pinion_stp_1_RIGID : Subsystem
  rack_stp_1_RIGID : Subsystem
  rack_stp_2_RIGID : Subsystem
  F : PMIOPort  Side=Right
  connections:
  Transform/RConn1 -- gripper_base_stp_1_RIGID/LConn1
  Transform1/RConn1 -- cube/LConn1 -- gripper_face_stp_1_RIGID/LConn1
  GRIPPER_ASM_0_stp_1_RIGID/LConn1 -- Transform14/RConn1
  ReferenceFrame/RConn1 -- Transform29/LConn1 -- Transform33/LConn1 -- Transform18/RConn1 -- Transform9/LConn1 -- RPi_Camera_V2_1_stp_1_RIGID/RConn1 -- Transform25/LConn1 -- Transform14/LConn1 -- Transform/LConn1 -- Transform1/LConn1
  Transform18/LConn1 -- F/RConn1
  SERVO_MOTOR_MICRO_9G_stp_1_RIGID/LConn1 -- Transform9/RConn1
  Transform33/RConn1 -- rack_stp_1_RIGID/LConn1
  Transform25/RConn1 -- rack_stp_2_RIGID/LConn1
  Transform29/RConn1 -- pinion_stp_1_RIGID/LConn1

== system ROBOTIC_ARM_sim/Robotic Arm/SERVO_MOTOR_MG996R_stp_1_RIGID ==
  ReferenceFrame : sm_lib/Frames and Transforms/Reference Frame
  Solid : sm_lib/Body Elements/File Solid  ExtGeomFileName=SERVO MOTOR MG996R.stp_Default_sldprt.STEP  UnitType=FromFile  ExtGeomFileUnits=m  StepReaderType=HEX  ExportConvexHullGeometry=off  InertiaType=Custom  BasedOnType=DensityFromFile  Density=1000  DensityUnits=kg/m^3  Mass=smiData.Solid(16).mass  MassUnits=kg  CenterOfMass=smiData.Solid(16).CoM  CenterOfMassUnits=mm  MomentsOfInertia=smiData.Solid(16).MoI  MomentsOfInertiaUnits=kg*mm^2  ProductsOfInertia=smiData.Solid(16).PoI  ProductsOfInertiaUnits=kg*mm^2  GraphicType=FromGeometry  MarkerShape=Sphere  MarkerSize=10  GraphicVisPropType=SimpleVisualProperties  GraphicDiffuseColor=[0.149 0.149 0.149]  GraphicOpacity=smiData.Solid(16).opacity  GraphicSpecularColor=[0.5 0.5 0.5 1.0]  GraphicAmbientColor=[0.15 0.15 0.15 1.0]  GraphicEmissiveColor=[0.0 0.0 0.0 1.0]  GraphicShininess=75  DoExposeReferenceFrame=on  SerializedFrames=<Frames/>
  F : PMIOPort  Side=Left
  connections:
  ReferenceFrame/RConn1 -- Solid/RConn1 -- F/RConn1

== system ROBOTIC_ARM_sim/Robotic Arm/SERVO_MOTOR_MG996R_stp_2_RIGID ==
  ReferenceFrame : sm_lib/Frames and Transforms/Reference Frame
  Solid : sm_lib/Body Elements/File Solid  ExtGeomFileName=SERVO MOTOR MG996R.stp_Default_sldprt.STEP  UnitType=FromFile  ExtGeomFileUnits=m  StepReaderType=HEX  ExportConvexHullGeometry=off  InertiaType=Custom  BasedOnType=DensityFromFile  Density=1000  DensityUnits=kg/m^3  Mass=smiData.Solid(16).mass  MassUnits=kg  CenterOfMass=smiData.Solid(16).CoM  CenterOfMassUnits=mm  MomentsOfInertia=smiData.Solid(16).MoI  MomentsOfInertiaUnits=kg*mm^2  ProductsOfInertia=smiData.Solid(16).PoI  ProductsOfInertiaUnits=kg*mm^2  GraphicType=FromGeometry  MarkerShape=Sphere  MarkerSize=10  GraphicVisPropType=SimpleVisualProperties  GraphicDiffuseColor=[0.149 0.149 0.149]  GraphicOpacity=smiData.Solid(16).opacity  GraphicSpecularColor=[0.5 0.5 0.5 1.0]  GraphicAmbientColor=[0.15 0.15 0.15 1.0]  GraphicEmissiveColor=[0.0 0.0 0.0 1.0]  GraphicShininess=75  DoExposeReferenceFrame=on  SerializedFrames=<Frames/>
  F : PMIOPort  Side=Left
  connections:
  ReferenceFrame/RConn1 -- Solid/RConn1 -- F/RConn1

== system ROBOTIC_ARM_sim/Robotic Arm/SERVO_MOTOR_MICRO_9G_stp_1_RIGID ==
  ReferenceFrame : sm_lib/Frames and Transforms/Reference Frame
  Solid : sm_lib/Body Elements/File Solid  ExtGeomFileName=SERVO MOTOR MICRO 9G.stp_Default_sldprt.STEP  UnitType=FromFile  ExtGeomFileUnits=m  StepReaderType=HEX  ExportConvexHullGeometry=off  InertiaType=Custom  BasedOnType=DensityFromFile  Density=1000  DensityUnits=kg/m^3  Mass=smiData.Solid(11).mass  MassUnits=kg  CenterOfMass=smiData.Solid(11).CoM  CenterOfMassUnits=mm  MomentsOfInertia=smiData.Solid(11).MoI  MomentsOfInertiaUnits=kg*mm^2  ProductsOfInertia=smiData.Solid(11).PoI  ProductsOfInertiaUnits=kg*mm^2  GraphicType=FromGeometry  MarkerShape=Sphere  MarkerSize=10  GraphicVisPropType=SimpleVisualProperties  GraphicDiffuseColor=[0.07451 0.6235 1]  GraphicOpacity=smiData.Solid(11).opacity  GraphicSpecularColor=[0.5 0.5 0.5 1.0]  GraphicAmbientColor=[0.15 0.15 0.15 1.0]  GraphicEmissiveColor=[0.0 0.0 0.0 1.0]  GraphicShininess=75  DoExposeReferenceFrame=on  SerializedFrames=<Frames/>
  F : PMIOPort  Side=Left
  connections:
  ReferenceFrame/RConn1 -- Solid/RConn1 -- F/RConn1

== system ROBOTIC_ARM_sim/Robotic Arm/WAIST_stp_1_RIGID ==
  ReferenceFrame : sm_lib/Frames and Transforms/Reference Frame
  Solid : sm_lib/Body Elements/File Solid  ExtGeomFileName=WAIST.stp_Default_sldprt.STEP  UnitType=FromFile  ExtGeomFileUnits=m  StepReaderType=HEX  ExportConvexHullGeometry=off  InertiaType=Custom  BasedOnType=DensityFromFile  Density=1000  DensityUnits=kg/m^3  Mass=smiData.Solid(14).mass  MassUnits=kg  CenterOfMass=smiData.Solid(14).CoM  CenterOfMassUnits=mm  MomentsOfInertia=smiData.Solid(14).MoI  MomentsOfInertiaUnits=kg*mm^2  ProductsOfInertia=smiData.Solid(14).PoI  ProductsOfInertiaUnits=kg*mm^2  GraphicType=FromGeometry  MarkerShape=Sphere  MarkerSize=10  GraphicVisPropType=SimpleVisualProperties  GraphicDiffuseColor=[1 1 0]  GraphicOpacity=smiData.Solid(14).opacity  GraphicSpecularColor=[0.5 0.5 0.5 1.0]  GraphicAmbientColor=[0.15 0.15 0.15 1.0]  GraphicEmissiveColor=[0.0 0.0 0.0 1.0]  GraphicShininess=75  DoExposeReferenceFrame=on  SerializedFrames=<Frames/>
  F : PMIOPort  Side=Left
  connections:
  Solid/RConn1 -- ReferenceFrame/RConn1 -- F/RConn1

== system ROBOTIC_ARM_sim/Robotic Arm/black_servo_extention_stp_1_RIGID ==
  ReferenceFrame : sm_lib/Frames and Transforms/Reference Frame
  Solid : sm_lib/Body Elements/File Solid  ExtGeomFileName=black servo extention.stp_Default_sldprt.STEP  UnitType=FromFile  ExtGeomFileUnits=m  StepReaderType=HEX  ExportConvexHullGeometry=off  InertiaType=Custom  BasedOnType=DensityFromFile  Density=1000  DensityUnits=kg/m^3  Mass=smiData.Solid(18).mass  MassUnits=kg  CenterOfMass=smiData.Solid(18).CoM  CenterOfMassUnits=mm  MomentsOfInertia=smiData.Solid(18).MoI  MomentsOfInertiaUnits=kg*mm^2  ProductsOfInertia=smiData.Solid(18).PoI  ProductsOfInertiaUnits=kg*mm^2  GraphicType=FromGeometry  MarkerShape=Sphere  MarkerSize=10  GraphicVisPropType=SimpleVisualProperties  GraphicDiffuseColor=[0.149 0.149 0.149]  GraphicOpacity=smiData.Solid(18).opacity  GraphicSpecularColor=[0.5 0.5 0.5 1.0]  GraphicAmbientColor=[0.15 0.15 0.15 1.0]  GraphicEmissiveColor=[0.0 0.0 0.0 1.0]  GraphicShininess=75  DoExposeReferenceFrame=on  SerializedFrames=<Frames/>
  F : PMIOPort  Side=Left
  connections:
  ReferenceFrame/RConn1 -- Solid/RConn1 -- F/RConn1

== system ROBOTIC_ARM_sim/Robotic Arm/black_servo_extention_stp_2_RIGID ==
  ReferenceFrame : sm_lib/Frames and Transforms/Reference Frame
  Solid : sm_lib/Body Elements/File Solid  ExtGeomFileName=black servo extention.stp_Default_sldprt.STEP  UnitType=FromFile  ExtGeomFileUnits=m  StepReaderType=HEX  ExportConvexHullGeometry=off  InertiaType=Custom  BasedOnType=DensityFromFile  Density=1000  DensityUnits=kg/m^3  Mass=smiData.Solid(18).mass  MassUnits=kg  CenterOfMass=smiData.Solid(18).CoM  CenterOfMassUnits=mm  MomentsOfInertia=smiData.Solid(18).MoI  MomentsOfInertiaUnits=kg*mm^2  ProductsOfInertia=smiData.Solid(18).PoI  ProductsOfInertiaUnits=kg*mm^2  GraphicType=FromGeometry  MarkerShape=Sphere  MarkerSize=10  GraphicVisPropType=SimpleVisualProperties  GraphicDiffuseColor=[0.149 0.149 0.149]  GraphicOpacity=smiData.Solid(18).opacity  GraphicSpecularColor=[0.5 0.5 0.5 1.0]  GraphicAmbientColor=[0.15 0.15 0.15 1.0]  GraphicEmissiveColor=[0.0 0.0 0.0 1.0]  GraphicShininess=75  DoExposeReferenceFrame=on  SerializedFrames=<Frames/>
  F : PMIOPort  Side=Left
  connections:
  ReferenceFrame/RConn1 -- Solid/RConn1 -- F/RConn1

== system ROBOTIC_ARM_sim/Robotic Arm/gripper_base_fixation_stp_1_RIGID ==
  ReferenceFrame : sm_lib/Frames and Transforms/Reference Frame
  Solid : sm_lib/Body Elements/File Solid  ExtGeomFileName=gripper base fixation.stp_Default_sldprt.STEP  UnitType=FromFile  ExtGeomFileUnits=m  StepReaderType=HEX  ExportConvexHullGeometry=off  InertiaType=Custom  BasedOnType=DensityFromFile  Density=1000  DensityUnits=kg/m^3  Mass=smiData.Solid(22).mass  MassUnits=kg  CenterOfMass=smiData.Solid(22).CoM  CenterOfMassUnits=mm  MomentsOfInertia=smiData.Solid(22).MoI  MomentsOfInertiaUnits=kg*mm^2  ProductsOfInertia=smiData.Solid(22).PoI  ProductsOfInertiaUnits=kg*mm^2  GraphicType=FromGeometry  MarkerShape=Sphere  MarkerSize=10  GraphicVisPropType=SimpleVisualProperties  GraphicDiffuseColor=[0.149 0.149 0.149]  GraphicOpacity=smiData.Solid(22).opacity  GraphicSpecularColor=[0.5 0.5 0.5 1.0]  GraphicAmbientColor=[0.15 0.15 0.15 1.0]  GraphicEmissiveColor=[0.0 0.0 0.0 1.0]  GraphicShininess=75  DoExposeReferenceFrame=on  SerializedFrames=<Frames/>
  F : PMIOPort  Side=Left
  connections:
  ReferenceFrame/RConn1 -- Solid/RConn1 -- F/RConn1

== system ROBOTIC_ARM_sim/Robotic Arm/link2_stp_1_RIGID ==
  ReferenceFrame : sm_lib/Frames and Transforms/Reference Frame
  Solid : sm_lib/Body Elements/File Solid  ExtGeomFileName=link2.stp_Default_sldprt.STEP  UnitType=FromFile  ExtGeomFileUnits=m  StepReaderType=HEX  ExportConvexHullGeometry=off  InertiaType=Custom  BasedOnType=DensityFromFile  Density=1000  DensityUnits=kg/m^3  Mass=smiData.Solid(17).mass  MassUnits=kg  CenterOfMass=smiData.Solid(17).CoM  CenterOfMassUnits=mm  MomentsOfInertia=smiData.Solid(17).MoI  MomentsOfInertiaUnits=kg*mm^2  ProductsOfInertia=smiData.Solid(17).PoI  ProductsOfInertiaUnits=kg*mm^2  GraphicType=FromGeometry  MarkerShape=Sphere  MarkerSize=10  GraphicVisPropType=SimpleVisualProperties  GraphicDiffuseColor=[1 1 0]  GraphicOpacity=smiData.Solid(17).opacity  GraphicSpecularColor=[0.5 0.5 0.5 1.0]  GraphicAmbientColor=[0.15 0.15 0.15 1.0]  GraphicEmissiveColor=[0.0 0.0 0.0 1.0]  GraphicShininess=75  DoExposeReferenceFrame=on  SerializedFrames=<Frames/>
  F : PMIOPort  Side=Left
  connections:
  ReferenceFrame/RConn1 -- Solid/RConn1 -- F/RConn1
